simulink model "projekt_mdl_3"  (R2009b)
settings: Solver=ode45  StartTime=0.0  StopTime=4  FixedStep=Ts  RelTol=1e-3
undefined symbols (not defined in the file): dGnf, dH_D, dId_g, dIq_g, DiscIntNeverNeededParam, dPLL, dQ, Lf, nGnf, nH_D, nId_g, nIq_g, nPLL, nQ, omega, plecs, Rd, Tds, Ts
libraries: simulink_extras x1
settings Model: Creator=Tomislav  LastModifiedBy=teja
settings DataIOCC: LimitDataPoints=on  SaveFormat=Array  SignalLoggingSaveFormat=ModelDataLogs  ReturnWorkspaceOutputs=off
settings OptimizationCC: ExpressionDepthLimit=2147483647  LifeSpan=inf  SimCompilerOptimization=Off
settings DebuggingCC: UnderspecifiedInitializationDetection=Classic  MergeDetectMultiDrivingBlocksExec=none  SolverPrmCheckMsg=warning  MultiTaskDSMMsg=warning  MultiTaskCondExecSysMsg=none  FcnCallInpInsideContextMsg=UseLocalSettings  FrameProcessingCompatibilityMsg=warning  StateNameClashWarn=warning  StrictBusMsg=None  SFUnexpectedBacktrackingDiag=warning  SFNoUnconditionalDefaultTransitionDiag=warning
settings HardwareCC: ProdBitPerPointer=32  ProdLargestAtomicFloat=None  ProdIntDivRoundTo=Undefined  ProdEndianess=Unspecified  ProdWordSize=32  ProdHWDeviceType=32-bit Generic
settings ModelReferenceCC: PropagateSignalLabelsOutOfModel=off
settings SFSimCC: SimUseLocalCustomCode=off
settings RTWCC: RTWUseLocalCustomCode=off  IncludeERTFirstTime=on  RTWCompilerOptimization=Off
settings GRTTargetCC: CodeReplacementLibrary=ANSI_C  GeneratePreprocessorConditionals=Disable all  CombineOutputUpdateFcns=off  CPPClassGenCompliant=off  GRTInterface=on

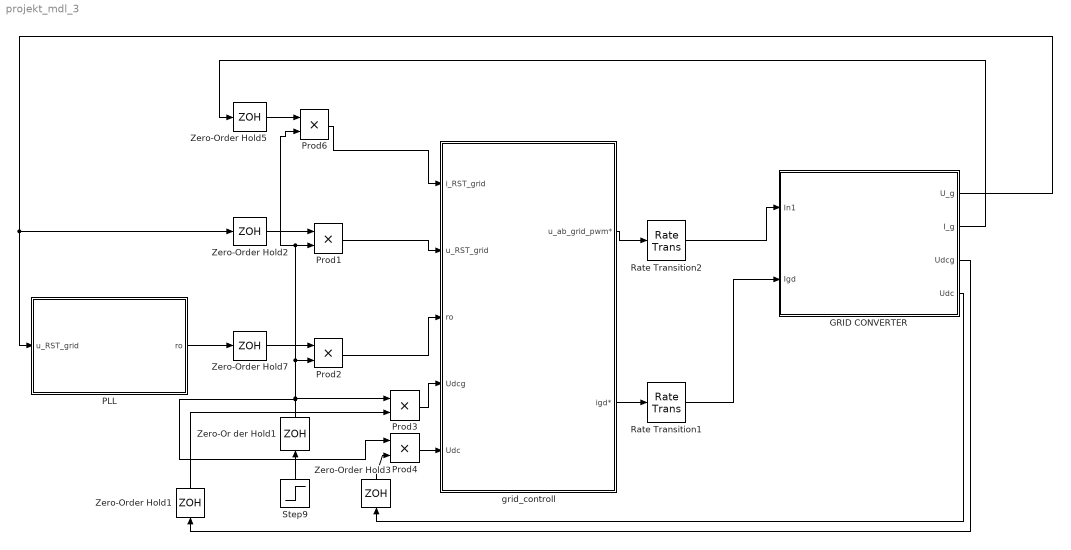
== system projekt_mdl_3 ==
  GRID CONVERTER : Subsystem  LoadFcn=plecs('sl', 200);  InitFcn=plecs('sl', 214);  StartFcn=plecs('sl', 208);  StopFcn=plecs('sl', 209);  mask(PlecsCircuit){PLECSData=<binary blob, 5148 chars, not shown>}
      mask prompts: PLECSData "PLECS Data (Do not delete or modify!)"
      mask init:
      | % PLACE CUSTOM INITIALIZATIONS ABOVE
      | % DO NOT REMOVE
      | plecs('sl', 215);
      | % DO NOT REMOVE
      settings: CopyFcn=plecs('sl', 203);  DeleteFcn=plecs('sl', 205);  UndoDeleteFcn=plecs('sl', 206);  PreSaveFcn=plecs('sl', 211);  PostSaveFcn=plecs('sl', 201);  NameChangeFcn=plecs('sl', 210);  DestroyFcn=plecs('sl', 207);  PreCopyFcn=plecs('sl', 216);  OpenFcn=plecs('sl', 202);  ErrorFcn=plerrorfcn
      mask Help: web(['file:///' fullfile(plecsdoc, 'creatingacircuit.html')])
      mask Display: disp('PLECS\nCircuit')
  PLL : Subsystem
  Prod{1..4,6} (5 alike) : Product  SampleTime=Tds
  Rate Transition1 : RateTransition  OutPortSampleTimeOpt=Inherit  OutPortSampleTime=Tds
  Rate Transition2 : RateTransition  OutPortSampleTimeOpt=Inherit  OutPortSampleTime=Tds
  Step9 : Step  Time=0.2  SampleTime=Ts
  Zero-Or der Hold1 : ZeroOrderHold  SampleTime=Tds
  Zero-Order Hold{1..3,5,7} (5 alike) : ZeroOrderHold  SampleTime=Tds
  grid_controll : Subsystem
  wires:
  Step9/1 -> Zero-Or der Hold1/1
  grid_controll/1("u_ab_grid_pwm* ") -> Rate Transition2/1
  Zero-Order Hold5/1 -> Prod6/1
  Prod1/1 -> grid_controll/2(u_RST_grid)
  Zero-Order Hold2/1 -> Prod1/1
  Prod2/1 -> grid_controll/3(ro)
  Zero-Order Hold7/1 -> Prod2/1
  PLL/1("ro ") -> Zero-Order Hold7/1
  Rate Transition2/1 -> GRID CONVERTER/1(In1)
  GRID CONVERTER/1(U_g) -> PLL/1(u_RST_grid), Zero-Order Hold2/1
  GRID CONVERTER/2(I_g) -> Zero-Order Hold5/1
  Prod6/1 -> grid_controll/1(i_RST_grid)
  GRID CONVERTER/3(Udcg) -> Zero-Order Hold1/1
  Zero-Order Hold1/1 -> Prod3/2
  Zero-Or der Hold1/1 -> Prod3/1, Prod6/2, Prod1/2, Prod2/2, Prod4/1
  Prod3/1 -> grid_controll/4(Udcg)
  GRID CONVERTER/4(Udc) -> Zero-Order Hold3/1
  Prod4/1 -> grid_controll/5(Udc)
  Zero-Order Hold3/1 -> Prod4/2
  grid_controll/2("igd* ") -> Rate Transition1/1
  Rate Transition1/1 -> GRID CONVERTER/2(Igd)

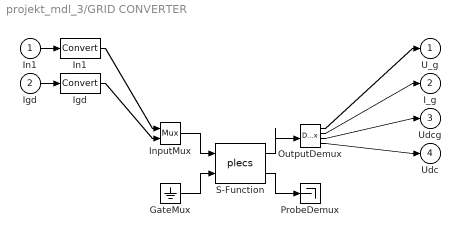
== system projekt_mdl_3/GRID CONVERTER ==
  In1 : Inport  PortDimensions=3
  Igd : Inport  Port=2  PortDimensions=1
  " GateMux " : Ground
  " Igd " : DataTypeConversion  SaturateOnIntegerOverflow=on  RndMeth=Zero
  " In1 " : DataTypeConversion  SaturateOnIntegerOverflow=on  RndMeth=Zero
  " InputMux " : Mux  Inputs=[ 3 1 ]
  " OutputDemux " : Demux  Outputs=[ 3 3 1 1 ]
  " ProbeDemux " : Terminator
  " S-Function " : S-Function  FunctionName=plecs  EnableBusSupport=off
  U_g : Outport  PortDimensions=3
  I_g : Outport  Port=2  PortDimensions=3
  Udcg : Outport  Port=3  PortDimensions=1
  Udc : Outport  Port=4  PortDimensions=1
  wires:
  " S-Function "/1 -> " OutputDemux "/1
  " InputMux "/1 -> " S-Function "/1
  " GateMux "/1 -> " S-Function "/2
  " S-Function "/2 -> " ProbeDemux "/1
  In1/1 -> " In1 "/1
  " In1 "/1 -> " InputMux "/1
  Igd/1 -> " Igd "/1
  " Igd "/1 -> " InputMux "/2
  " OutputDemux "/1 -> U_g/1
  " OutputDemux "/2 -> I_g/1
  " OutputDemux "/3 -> Udcg/1
  " OutputDemux "/4 -> Udc/1

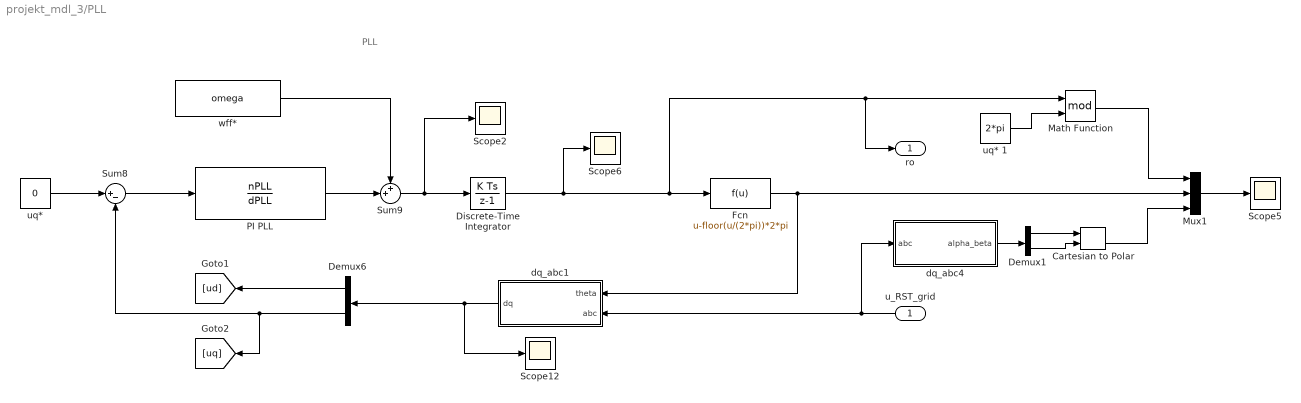
== system projekt_mdl_3/PLL ==
  note: PLL
  u_RST_grid : Inport
  Cartesian to Polar : simulink_extras/Transformations/Cartesian to Polar
  Demux1 : Demux  Outputs=2
  Demux6 : Demux  Outputs=2
  Discrete-Time Integrator : DiscreteIntegrator  SampleTime=Ts  ICPrevOutput=DiscIntNeverNeededParam  ICPrevScaledInput=DiscIntNeverNeededParam
  Fcn : Fcn  Expr=u-floor(u/(2*pi))*2*pi
  Math Function : Math  Operator=mod  SaturateOnIntegerOverflow=on
  Mux1 : Mux  Inputs=3
      settings: DisplayOption=signals
  PI PLL : DiscreteTransferFcn  Numerator=nPLL  Denominator=dPLL  SampleTime=Ts  a0EqualsOne=on
  Scope{2,5..6,12} (4 alike) : Scope
      Scope12 settings: YMin=648.75  YMax=649.65  SaveName=ScopeData9
      Scope2 settings: YMin=-329.867  YMax=-298.451  SaveName=ScopeData10
      Scope5 settings: YMin=-3.5  YMax=6.5  SaveName=ScopeData11
      Scope6 settings: YMin=-1056  YMax=-1045.5  SaveName=ScopeData12
  Sum8 : Sum  Inputs=|+-
  Sum9 : Sum  Inputs=++|
  dq_abc1 : Subsystem
  dq_abc4 : Subsystem
  "uq* " : Constant  Value=0
  uq* 1 : Constant  Value=2*pi
  "wff* " : Constant  Value=omega
  "ro " : Outport
  wires:
  "uq* "/1 -> Sum8/1
  Sum8/1 -> PI PLL/1
  PI PLL/1 -> Sum9/2
  Sum9/1 -> Scope2/1, Discrete-Time Integrator/1
  "wff* "/1 -> Sum9/1
  dq_abc1/1(dq) -> Scope12/1, Demux6/1
  Demux6/2 -> [uq], Sum8/2
  Demux6/1 -> [ud]
  Mux1/1 -> Scope5/1
  dq_abc4/1(alpha_beta) -> Demux1/1
  Demux1/1 -> Cartesian to Polar/1
  Demux1/2 -> Cartesian to Polar/2
  u_RST_grid/1 -> dq_abc1/2(abc), dq_abc4/1(abc)
  Discrete-Time Integrator/1 -> Fcn/1, Math Function/1, "ro "/1, Scope6/1
  Fcn/1 -> dq_abc1/1(theta), Mux1/2
  uq* 1/1 -> Math Function/2
  Math Function/1 -> Mux1/1
  Cartesian to Polar/2 -> Mux1/3

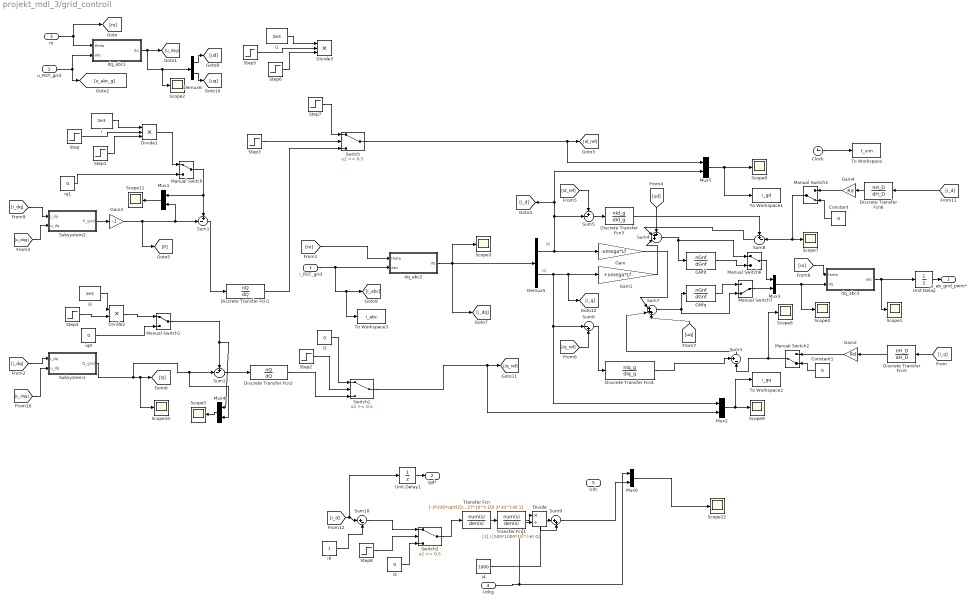
== system projekt_mdl_3/grid_controll ==
  note: iq
  note: id
  i_RST_grid : Inport  SampleTime=Ts
  u_RST_grid : Inport  Port=2
  ro : Inport  Port=3
  Udcg : Inport  Port=4
  Udc : Inport  Port=5
  Clock : Clock
  Constant : Constant  Value=0
  Constant1 : Constant  Value=0
  Demux5 : Demux  Outputs=2
  Demux6 : Demux  Outputs=2
  Discrete Transfer Fcn1 : DiscreteTransferFcn  Numerator=nQ  Denominator=dQ  SampleTime=Tds
  Discrete Transfer Fcn2 : DiscreteTransferFcn  Numerator=nQ  Denominator=dQ  SampleTime=Tds
  Discrete Transfer Fcn3 : DiscreteTransferFcn  Numerator=nId_g  Denominator=dId_g  SampleTime=Tds
  Discrete Transfer Fcn4 : DiscreteTransferFcn  Numerator=nIq_g  Denominator=dIq_g  SampleTime=Tds
  Discrete Transfer Fcn5 : DiscreteTransferFcn  Numerator=nH_D  Denominator=dH_D  SampleTime=Tds
  Discrete Transfer Fcn6 : DiscreteTransferFcn  Numerator=nH_D  Denominator=dH_D  SampleTime=Tds
  Divide : Product  Inputs=*/
  Divide1 : Product  Inputs=***  SampleTime=Tds
  Divide2 : Product  Inputs=**  SampleTime=Tds
  Divide3 : Product  Inputs=***  SampleTime=Tds
  GNfd : DiscreteTransferFcn  Numerator=nGnf  Denominator=dGnf  SampleTime=Tds
  GNfq : DiscreteTransferFcn  Numerator=nGnf  Denominator=dGnf  SampleTime=Tds
  Gain : Gain  Gain=-omega*Lf  SampleTime=Tds
  Gain1 : Gain  Gain=+omega*Lf  SampleTime=Tds
  Gain2 : Gain  Gain=Rd  SampleTime=Tds
  Gain3 : Gain  Gain=-1
  Gain4 : Gain  Gain=Rd  SampleTime=Tds
  Manual Switch : ManualSwitch
  Manual Switch1 : ManualSwitch
  Manual Switch2 : ManualSwitch  CurrentSetting=0
  Manual Switch3 : ManualSwitch  CurrentSetting=0
  Manual Switch6 : ManualSwitch
  Manual Switch7 : ManualSwitch  CurrentSetting=0
  Mux{1..6} (6 alike) : Mux  Inputs=2
      Mux1 settings: DisplayOption=signals
      Mux2 settings: DisplayOption=signals
      Mux4 settings: DisplayOption=signals
      Mux5 settings: DisplayOption=signals
  Scope{1..12} (12 alike) : Scope
      Scope1 settings: YMin=-7e+15  YMax=7e+15  SaveName=ScopeData16
      Scope10 settings: YMin=-17.5  YMax=2.5  SaveName=ScopeData4
      Scope11 settings: YMin=-17.5  YMax=2.5  SaveName=Pdata
      Scope12 settings: YMin=380  YMax=600  SaveName=ScopeData3
      Scope2 settings: YMin=-17.5  YMax=2.5
      Scope3 settings: YMin=-17.5  YMax=2.5  SaveName=ScopeData22
      Scope4 settings: YMin=-0.5  YMax=10.5  SaveName=ScopeData23
      Scope5 settings: YMin=-17.5  YMax=2.5  SaveName=Qdata
      Scope6 settings: YMin=-250  YMax=250
      Scope7 settings: YMin=-300  YMax=300  SaveName=ScopeData2
      Scope8 settings: TimeRange=1  YMin=-350  YMax=75  SaveName=Iddata
      Scope9 settings: TimeRange=3  YMin=-800000  YMax=600000  SaveName=Iqdata
  Step : Step  SampleTime=Tds
  Step1 : Step  Time=2.5  Before=1  After=3/2  SampleTime=Tds
  Step2 : Step  Time=0.5  SampleTime=Tds
  Step3 : Step  Time=0.5  SampleTime=Tds
  Step4 : Step  SampleTime=Tds
  Step5 : Step  SampleTime=Tds
  Step6 : Step  Time=2.5  Before=1  After=3/2  SampleTime=Tds
  Step7 : Step  Time=2  Before=1  SampleTime=Tds
  Step8 : Step  Time=3  SampleTime=Tds
  Subsystem1 : Subsystem
  Subsystem2 : Subsystem
  Sum{1..3,5,8} (5 alike) : Sum  Inputs=+-|  SampleTime=Tds
  Sum10 : Sum  Inputs=|+-  SampleTime=Tds
  Sum4 : Sum  Inputs=+++|  SampleTime=Tds
  Sum6 : Sum  Inputs=|-+  SampleTime=Tds
  Sum7 : Sum  Inputs=|+++  SampleTime=Tds
  Sum9 : Sum  Inputs=|++  SampleTime=Tds
  Switch : Switch  Threshold=0.5
  Switch1 : Switch  Threshold=0.5
  Switch2 : Switch  Threshold=0.5
  To Workspace : ToWorkspace  VariableName=t_sim  SampleTime=-1
  To Workspace1 : ToWorkspace  VariableName=i_gd  SampleTime=-1
  To Workspace2 : ToWorkspace  VariableName=i_gq  SampleTime=-1
  To Workspace3 : ToWorkspace  VariableName=i_abc  SampleTime=Tds
  Transfer Fcn : TransferFcn  Numerator=[-3*230*sqrt(2)/4]  Denominator=[2.27*10^(-10) 3*10^(-8) 1]
  Transfer Fcn1 : TransferFcn  Denominator=[500*1000*10^(-6) 0]
  Unit Delay : UnitDelay  SampleTime=Tds
  Unit Delay1 : UnitDelay  SampleTime=Tds
  dq_abc1 : Subsystem
  dq_abc2 : Subsystem
  dq_abc3 : Subsystem
  i : Constant  Value=2e3  SampleTime=Tds
  i1 : Constant  Value=2e3  SampleTime=Tds
  i2 : Constant  Value=0
  i3 : Constant  Value=1e3  SampleTime=Tds
  i4 : Constant  Value=1000
  i5 : Constant  Value=0
  i6 : Constant
  iq0 : Constant  Value=0
  iq1 : Constant  Value=0
  "u_ab_grid_pwm* " : Outport
  "igd* " : Outport  Port=2
  wires:
  Demux5/1 -> Gain/1, Sum5/2, [i_d], Mux5/2
  [ud] -> Sum4/1
  [id_ref] -> Sum5/1
  Sum5/1 -> Discrete Transfer Fcn3/1
  [ro] -> dq_abc3/1(theta)
  [ro] -> dq_abc2/1(theta)
  dq_abc2/1(dq) -> [i_dq], Scope3/1, Demux5/1
  dq_abc3/1("abc ") -> Unit Delay/1, Scope1/1
  Mux5/1 -> To Workspace1/1, Scope8/1
  i_RST_grid/1 -> dq_abc2/2(abc), To Workspace3/1, [i_abc]
  Mux2/1 -> To Workspace2/1, Scope9/1
  Demux5/2 -> Sum6/1, Mux2/1, [i_q], Gain1/1
  ro/1 -> [ro], dq_abc1/1(theta)
  u_RST_grid/1 -> dq_abc1/2(abc), [u_abc_g]
  dq_abc1/1(dq) -> Scope2/1, Demux6/1, [u_dqg]
  Demux6/1 -> [ud]
  Demux6/2 -> [uq]
  Clock/1 -> To Workspace/1
  Switch1/1 -> Mux2/2, [iq_ref]
  i/1 -> Divide1/1
  Step/1 -> Divide1/2
  Step1/1 -> Divide1/3
  Divide1/1 -> Manual Switch/1
  [iq_ref] -> Sum6/2
  Unit Delay/1 -> "u_ab_grid_pwm* "/1
  Gain/1 -> Sum7/1
  Gain1/1 -> Sum4/3
  [uq] -> Sum7/3
  Sum6/1 -> Discrete Transfer Fcn4/1
  [i_dq] -> Subsystem1/1(i_dq)
  Subsystem1/1("Q_grid ") -> [Q], Scope10/1, Sum2/2, Mux4/2
  [u_dqg] -> Subsystem1/2(u_dq)
  Sum1/1 -> Discrete Transfer Fcn1/1
  Switch/1 -> [id_ref], Mux5/1
  Step3/1 -> Switch/2
  [i_dq] -> Subsystem2/1(i_dq)
  [u_dqg] -> Subsystem2/2(u_dq)
  Discrete Transfer Fcn1/1 -> Switch/3
  Subsystem2/1(P_grid) -> Gain3/1
  Mux1/1 -> Scope11/1
  Gain3/1 -> Sum1/2, Mux1/2, [P]
  iq0/1 -> Manual Switch1/2
  Sum2/1 -> Discrete Transfer Fcn2/1
  Discrete Transfer Fcn2/1 -> Switch1/3
  Step2/1 -> Switch1/2
  i2/1 -> Switch1/1
  Mux4/1 -> Scope5/1
  iq1/1 -> Manual Switch/2
  Manual Switch/1 -> Sum1/1, Mux1/1
  i3/1 -> Divide2/1
  Step4/1 -> Divide2/2
  Divide2/1 -> Manual Switch1/1
  Manual Switch1/1 -> Sum2/1, Mux4/1
  i1/1 -> Divide3/1
  Step5/1 -> Divide3/2
  Step6/1 -> Divide3/3
  Step7/1 -> Switch/1
  Mux3/1 -> Scope4/1, dq_abc3/2(dq)
  [i_q] -> Discrete Transfer Fcn5/1
  [i_d] -> Discrete Transfer Fcn6/1
  Manual Switch2/1 -> Scope6/1, Sum3/2
  Manual Switch3/1 -> Sum8/2, Scope7/1
  Constant/1 -> Manual Switch3/2
  Constant1/1 -> Manual Switch2/2
  Sum4/1 -> Manual Switch6/1, GNfd/1
  Sum8/1 -> Sum4/2
  Sum7/1 -> GNfq/1, Manual Switch7/2
  Sum3/1 -> Sum7/2
  Discrete Transfer Fcn5/1 -> Gain2/1
  Discrete Transfer Fcn6/1 -> Gain4/1
  Discrete Transfer Fcn4/1 -> Sum3/1
  Discrete Transfer Fcn3/1 -> Sum8/1
  Gain2/1 -> Manual Switch2/1
  Gain4/1 -> Manual Switch3/1
  GNfd/1 -> Manual Switch6/2
  Manual Switch6/1 -> Mux3/1
  Manual Switch7/1 -> Mux3/2
  GNfq/1 -> Manual Switch7/1
  Udcg/1 -> Divide/2, Mux6/1
  Mux6/1 -> Scope12/1
  Transfer Fcn/1 -> Transfer Fcn1/1
  Sum9/1 -> Mux6/2
  i4/1 -> Sum9/2
  Step8/1 -> Switch2/2
  i5/1 -> Switch2/3
  Transfer Fcn1/1 -> Divide/1
  Divide/1 -> Sum9/1
  Switch2/1 -> Transfer Fcn/1
  i6/1 -> Sum10/2
  Sum10/1 -> Switch2/1
  [i_d] -> Unit Delay1/1, Sum10/1
  Unit Delay1/1 -> "igd* "/1

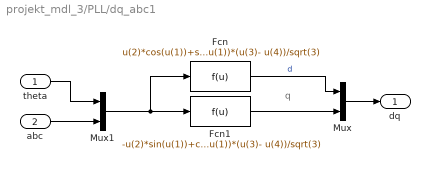
== system projekt_mdl_3/PLL/dq_abc1 ==
  note: q
  theta : Inport
  abc : Inport  Port=2
  Fcn : Fcn  Expr=u(2)*cos(u(1))+sin(u(1))*(u(3)- u(4))/sqrt(3)
  Fcn1 : Fcn  Expr=-u(2)*sin(u(1))+cos(u(1))*(u(3)- u(4))/sqrt(3)
  Mux : Mux  Inputs=2
  Mux1 : Mux  Inputs=2
  dq : Outport
  wires:
  abc/1 -> Mux1/2
  theta/1 -> Mux1/1
  Fcn1/1 -> Mux/2
  Mux/1 -> dq/1
  Fcn/1 -> Mux/1  "d"
  Mux1/1 -> Fcn1/1, Fcn/1

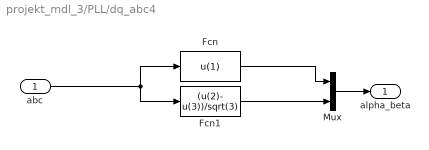
== system projekt_mdl_3/PLL/dq_abc4 ==
  abc : Inport
  Fcn : Fcn  Expr=u(1)
  Fcn1 : Fcn  Expr=(u(2)- u(3))/sqrt(3)
  Mux : Mux  Inputs=2
  alpha_beta : Outport
  wires:
  abc/1 -> Fcn1/1, Fcn/1
  Fcn/1 -> Mux/1
  Mux/1 -> alpha_beta/1
  Fcn1/1 -> Mux/2

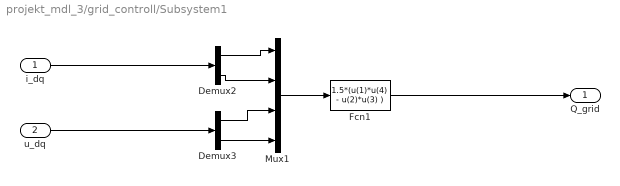
== system projekt_mdl_3/grid_controll/Subsystem1 ==
  i_dq : Inport
  u_dq : Inport  Port=2
  Demux2 : Demux  Outputs=2
  Demux3 : Demux  Outputs=2
  Fcn1 : Fcn  Expr=1.5*(u(1)*u(4) - u(2)*u(3) )
  Mux1 : Mux
  "Q_grid " : Outport
  wires:
  Demux3/2 -> Mux1/4
  Demux3/1 -> Mux1/3
  u_dq/1 -> Demux3/1
  i_dq/1 -> Demux2/1
  Fcn1/1 -> "Q_grid "/1
  Mux1/1 -> Fcn1/1
  Demux2/2 -> Mux1/2
  Demux2/1 -> Mux1/1

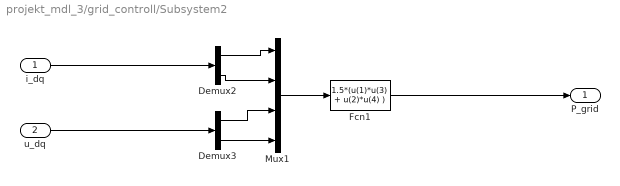
== system projekt_mdl_3/grid_controll/Subsystem2 ==
  i_dq : Inport
  u_dq : Inport  Port=2
  Demux2 : Demux  Outputs=2
  Demux3 : Demux  Outputs=2
  Fcn1 : Fcn  Expr=1.5*(u(1)*u(3) + u(2)*u(4) )
  Mux1 : Mux
  P_grid : Outport
  wires:
  Demux3/2 -> Mux1/4
  Demux3/1 -> Mux1/3
  u_dq/1 -> Demux3/1
  i_dq/1 -> Demux2/1
  Fcn1/1 -> P_grid/1
  Mux1/1 -> Fcn1/1
  Demux2/2 -> Mux1/2
  Demux2/1 -> Mux1/1

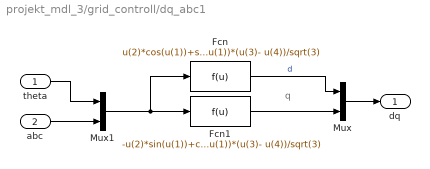
== system projekt_mdl_3/grid_controll/dq_abc1 ==
  note: q
  theta : Inport
  abc : Inport  Port=2
  Fcn : Fcn  Expr=u(2)*cos(u(1))+sin(u(1))*(u(3)- u(4))/sqrt(3)  SampleTime=Tds
  Fcn1 : Fcn  Expr=-u(2)*sin(u(1))+cos(u(1))*(u(3)- u(4))/sqrt(3)  SampleTime=Tds
  Mux : Mux  Inputs=2
  Mux1 : Mux  Inputs=2
  dq : Outport
  wires:
  Mux1/1 -> Fcn/1, Fcn1/1
  Fcn/1 -> Mux/1  "d"
  Mux/1 -> dq/1
  Fcn1/1 -> Mux/2
  theta/1 -> Mux1/1
  abc/1 -> Mux1/2

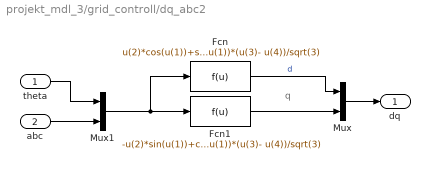
== system projekt_mdl_3/grid_controll/dq_abc2 ==
  note: q
  theta : Inport
  abc : Inport  Port=2
  Fcn : Fcn  Expr=u(2)*cos(u(1))+sin(u(1))*(u(3)- u(4))/sqrt(3)  SampleTime=Tds
  Fcn1 : Fcn  Expr=-u(2)*sin(u(1))+cos(u(1))*(u(3)- u(4))/sqrt(3)  SampleTime=Tds
  Mux : Mux  Inputs=2
  Mux1 : Mux  Inputs=2
  dq : Outport
  wires:
  Mux1/1 -> Fcn/1, Fcn1/1
  Fcn/1 -> Mux/1  "d"
  Mux/1 -> dq/1
  Fcn1/1 -> Mux/2
  theta/1 -> Mux1/1
  abc/1 -> Mux1/2

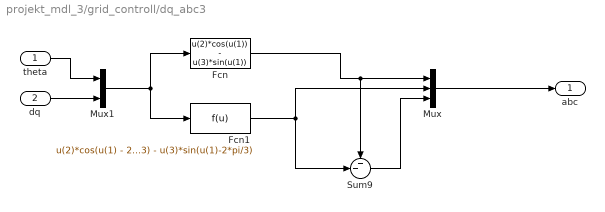
== system projekt_mdl_3/grid_controll/dq_abc3 ==
  theta : Inport
  dq : Inport  Port=2
  Fcn : Fcn  Expr=u(2)*cos(u(1)) - u(3)*sin(u(1))
  Fcn1 : Fcn  Expr=u(2)*cos(u(1) - 2*pi/3) - u(3)*sin(u(1)-2*pi/3)
  Mux : Mux  Inputs=3
  Mux1 : Mux  Inputs=2
  Sum9 : Sum  Inputs=--|
  "abc " : Outport
  wires:
  dq/1 -> Mux1/2
  theta/1 -> Mux1/1
  Mux/1 -> "abc "/1
  Fcn/1 -> Mux/1, Sum9/1
  Mux1/1 -> Fcn1/1, Fcn/1
  Fcn1/1 -> Mux/2, Sum9/2
  Sum9/1 -> Mux/3
